simulink model "RA5_student"  (R2015b)
settings: Solver=ode1  StartTime=0.0  StopTime=1000  FixedStep=1/(1024*4)  RelTol=1e-3
settings Model: SimulationMode=external  Creator=root  LastModifiedBy=root
settings DataIOCC: LimitDataPoints=off  SaveFormat=Array  SignalLoggingSaveFormat=ModelDataLogs
settings OptimizationCC: ExpressionDepthLimit=2147483647  InitFltsAndDblsToZero=on
settings DebuggingCC: UnderspecifiedInitializationDetection=Classic  MergeDetectMultiDrivingBlocksExec=none  FcnCallInpInsideContextMsg=UseLocalSettings  UnconnectedInputMsg=none  UnconnectedOutputMsg=none  UnconnectedLineMsg=none  StateNameClashWarn=warning
settings HardwareCC: ProdBitPerPointer=32  ProdLargestAtomicFloat=None  ProdIntDivRoundTo=Undefined  ProdEndianess=Unspecified  ProdWordSize=32  ProdHWDeviceType=32-bit Generic
settings RTWCC: SystemTargetFile=ectarget.tlc  MakeCommand="make_rtw OPTS=\"-DNETIF_ID=2\""  TemplateMakefile=ec_unix.tmf  Description=EtherCAT Real-Time Target for SOEM  RTWVerbose=off  CustomInclude=/home/ebox/MATLAB/R2015b/toolbox/shapeit/
settings RTWCC: CustomSource=|
  | /home/ebox/MATLAB/R2015b/toolbox/shapeit/dleadlag.c
  | /home/ebox/MATLAB/R2015b/toolbox/shapeit/dlowpass2.c
  | /home/ebox/MATLAB/R2015b/toolbox/shapeit/dnotch.c
  | /home/ebox/MATLAB/R2015b/toolbox/shapeit/dpd.c
  | /home/ebox/MATLAB/R2015b/toolbox/shapeit/dweakint.c
settings GRTTargetCC: GeneratePreprocessorConditionals=Disable all  CombineOutputUpdateFcns=off  GRTInterface=on  UseToolchainInfoCompliant=off  ExtMode=on
settings ConfigComp: CovModelRefEnable=Off

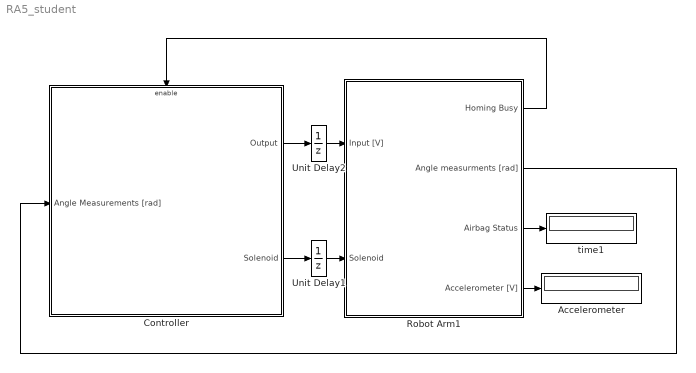
== system RA5_student ==
  Accelerometer : Display
      settings: Decimation=50
  Controller : Subsystem
  Robot Arm1 : Subsystem
      mask help: Simulink:masks:GenSFuncDesc_MD
      mask Help: eval('feval(''rtwprivate'',''rtwhelpview'',''rtw_sfcn_block'')');
      mask Display:
      | image(imread('RobotArm.png'))
      | color('red');port_label('output', 1, 'Homing Busy')
      | port_label('output', 2, 'Angle Measurements')
      | port_label('output', 3, 'Airbag Status')
      | port_label('output', 4, 'Accelerometer [V]')
      | port_label('input', 1, 'Input [V]')
      | port_label('input', 2, 'Solenoid')
  Unit Delay1 : UnitDelay  SampleTime=-1
  Unit Delay2 : UnitDelay  SampleTime=-1
  time1 : Display
      settings: Decimation=50
  wires:
  Controller/1(Output) -> Unit Delay2/1
  Robot Arm1/1(Homing Busy) -> Controller/Enable
  Robot Arm1/2(Angle measurments [rad]) -> Controller/1(Angle Measurements [rad])
  Robot Arm1/3(Airbag Status) -> time1/1
  Controller/2(Solenoid) -> Unit Delay1/1
  Robot Arm1/4(Accelerometer [V]) -> Accelerometer/1
  Unit Delay2/1 -> Robot Arm1/1(Input [V])
  Unit Delay1/1 -> Robot Arm1/2(Solenoid)

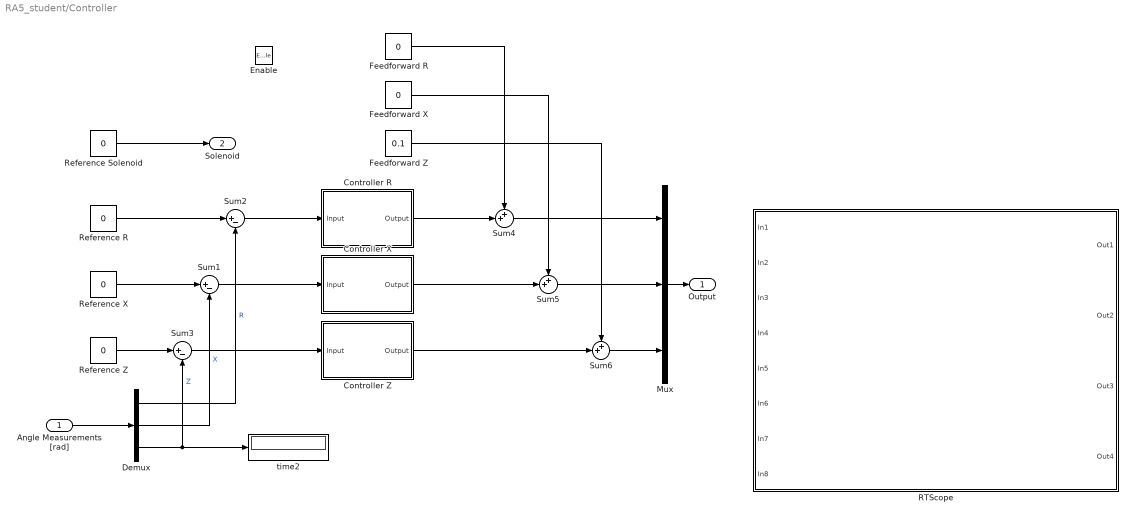
== system RA5_student/Controller ==
  Angle Measurements [rad] : Inport
  Enable : EnablePort
  Controller R : Subsystem
  Controller X : Subsystem
  Controller Z : Subsystem
  Demux : Demux  Outputs=3
  Feedforward R : Constant  Value=0
  Feedforward X : Constant  Value=0
  Feedforward Z : Constant  Value=0.1
  Mux : Mux  Inputs=3
  RTScope : Subsystem  mask(RTScope){}
      settings: OpenFcn=rtscope
      mask Display: image(imread('rtscope2.jpg'))
  Reference R : Constant  Value=0
  Reference Solenoid : Constant  Value=0
  Reference X : Constant  Value=0
  Reference Z : Constant  Value=0
  Sum1 : Sum  Inputs=|+-
  Sum2 : Sum  Inputs=|+-
  Sum3 : Sum  Inputs=|+-
  Sum4 : Sum  Inputs=++|  SaturateOnIntegerOverflow=on  InputSameDT=on  OutDataTypeStr=Inherit: Same as first input
  Sum5 : Sum  Inputs=++|  SaturateOnIntegerOverflow=on  InputSameDT=on  OutDataTypeStr=Inherit: Same as first input
  Sum6 : Sum  Inputs=++|  SaturateOnIntegerOverflow=on  InputSameDT=on  OutDataTypeStr=Inherit: Same as first input
  time2 : Display
      settings: Decimation=50
  Output : Outport
  Solenoid : Outport  Port=2  InitialOutput=0
  wires:
  Mux/1 -> Output/1
  Angle Measurements [rad]/1 -> Demux/1
  Sum2/1 -> Controller R/1(Input)
  Sum3/1 -> Controller Z/1(Input)
  Sum1/1 -> Controller X/1(Input)
  Demux/1 -> Sum2/2  "R"
  Demux/2 -> Sum1/2  "X"
  Demux/3 -> Sum3/2, time2/1  "Z"
  Feedforward R/1 -> Sum4/1
  Controller R/1(Output) -> Sum4/2
  Sum4/1 -> Mux/1
  Feedforward X/1 -> Sum5/1
  Controller X/1(Output) -> Sum5/2
  Sum5/1 -> Mux/2
  Controller Z/1(Output) -> Sum6/2
  Sum6/1 -> Mux/3
  Feedforward Z/1 -> Sum6/1
  Reference R/1 -> Sum2/1
  Reference X/1 -> Sum1/1
  Reference Z/1 -> Sum3/1
  Reference Solenoid/1 -> Solenoid/1

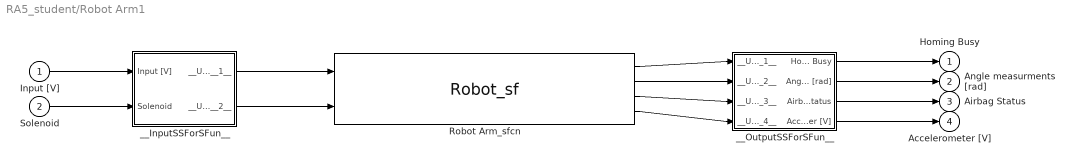
== system RA5_student/Robot Arm1 ==
  Input [V] : Inport
  Solenoid : Inport  Port=2
  Robot Arm_sfcn : S-Function  FunctionName=Robot_sf  SFunctionModules=dlowpass2 dnotch dpd dweakint ec_Ebox ec_EboxResetEnc  SFunctionDeploymentMode=off  EnableBusSupport=off  mask{rtw_sf_name=Robot_sf, showVar=off}
      mask prompts: rtw_sf_name "Simulink:masks:GenSFuncName_MP"; showVar "Simulink:masks:GenSFuncShowModuleList_MP"
      mask help: Simulink:masks:GenSFuncDesc_MD
      mask init:
      | displist = '';
      | if ~strcmp(get_param(gcb, 'FunctionName'), rtw_sf_name);
      |   set_param(gcb, 'FunctionName', rtw_sf_name);
      | end
      | % Check if we are generating code
      | rtw_mode = false;
      | if strcmpi(get_param(bdroot(gcb),'SimulationStatus'),'Initializing')
      | 	rtw_mode = strcmpi(get_param(bdroot(gcb),'BuildingRTWCode'),'on') && ...
      | 		~strcmpi(get_param(bdroot(gcb),'TargetStyle'),'SimulationTarget');
      | end
      | if showVar || rtw_mode
      | 	if exist('rtwsfunc') == 2 | exist('rtwsfunc') == 6
      | 		tmplist = rtwsfunc(rtw_sf_name,gcb);
      | 		tmplist = DAStudio.message('Simulink:masks:GenSFuncListOfModules_IC', tmplist);
      | 	elseif showVar
      | 		tmplist1 = DAStudio.message('Simulink:masks:GenSFuncListOfModules_IC', '');
      |         tmplist2 = DAStudio.message('Simulink:masks:GenSFuncNotLicensed_IC');
      |         tmplist = [tmplist1 tmplist2];
      |  	end
      | end
      | if showVar
      |   displist = tmplist;
      | end
      settings: CopyFcn=|
      | if ~strcmp(get_param(gcb,'Linkstatus'),'none') && ...
      | ~strcmp(get_param(gcb,'Linkstatus'),'implicit')
      |   set_param(gcb,'LinkStatus','none');
      | end
      mask Help: eval('feval(''rtwprivate'',''rtwhelpview'',''rtw_sfcn_block'')');
      mask Display:
      | port_label('input',1,'Input [V]');
      | port_label('input',2,'Solenoid');
      | port_label('output',1,'Homing Busy');
      | port_label('output',2,'Angle measurments [rad]');
      | port_label('output',3,'Airbag Status');
      | port_label('output',4,'Accelerometer [V]');
  __InputSSForSFun__ : Subsystem
  __OutputSSForSFun__ : Subsystem
  Homing Busy : Outport
  Angle measurments [rad] : Outport  Port=2
  Airbag Status : Outport  Port=3
  Accelerometer [V] : Outport  Port=4
  wires:
  __OutputSSForSFun__/4(Accelerometer [V]) -> Accelerometer [V]/1
  __OutputSSForSFun__/3(Airbag Status) -> Airbag Status/1
  __OutputSSForSFun__/2(Angle measurments [rad]) -> Angle measurments [rad]/1
  __OutputSSForSFun__/1(Homing Busy) -> Homing Busy/1
  Robot Arm_sfcn/4 -> __OutputSSForSFun__/4(__UniqueInportName__4__)
  Robot Arm_sfcn/3 -> __OutputSSForSFun__/3(__UniqueInportName__3__)
  Robot Arm_sfcn/2 -> __OutputSSForSFun__/2(__UniqueInportName__2__)
  Robot Arm_sfcn/1 -> __OutputSSForSFun__/1(__UniqueInportName__1__)
  __InputSSForSFun__/2(__UniqueOutportName__2__) -> Robot Arm_sfcn/2
  __InputSSForSFun__/1(__UniqueOutportName__1__) -> Robot Arm_sfcn/1
  Solenoid/1 -> __InputSSForSFun__/2(Solenoid)
  Input [V]/1 -> __InputSSForSFun__/1(Input [V])

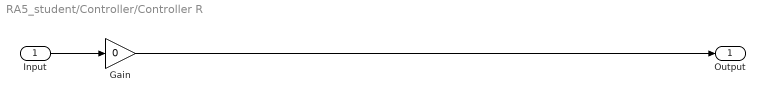
== system RA5_student/Controller/Controller R ==
  Input : Inport
  Gain : Gain  Gain=0
  Output : Outport
  wires:
  Input/1 -> Gain/1
  Gain/1 -> Output/1

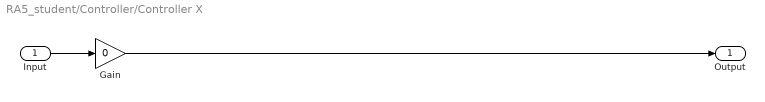
== system RA5_student/Controller/Controller X ==
  Input : Inport
  Gain : Gain  Gain=0
  Output : Outport
  wires:
  Gain/1 -> Output/1
  Input/1 -> Gain/1

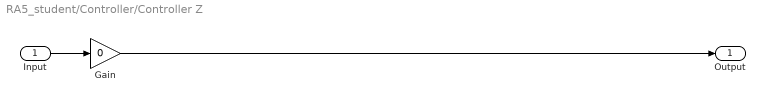
== system RA5_student/Controller/Controller Z ==
  Input : Inport
  Gain : Gain  Gain=0
  Output : Outport
  wires:
  Input/1 -> Gain/1
  Gain/1 -> Output/1

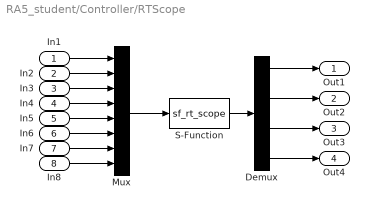
== system RA5_student/Controller/RTScope ==
  In1 : Inport
  In2 : Inport  Port=2
  In3 : Inport  Port=3
  In4 : Inport  Port=4
  In5 : Inport  Port=5
  In6 : Inport  Port=6
  In7 : Inport  Port=7
  In8 : Inport  Port=8
  Demux : Demux
  Mux : Mux  Inputs=8
  S-Function : S-Function  FunctionName=sf_rt_scope  Parameters=4096  SFunctionDeploymentMode=off  EnableBusSupport=off
  Out1 : Outport
  Out2 : Outport  Port=2
  Out3 : Outport  Port=3
  Out4 : Outport  Port=4
  wires:
  In8/1 -> Mux/8
  In7/1 -> Mux/7
  In6/1 -> Mux/6
  In5/1 -> Mux/5
  In4/1 -> Mux/4
  In3/1 -> Mux/3
  In2/1 -> Mux/2
  In1/1 -> Mux/1
  Demux/4 -> Out4/1
  Demux/3 -> Out3/1
  Demux/2 -> Out2/1
  Demux/1 -> Out1/1
  S-Function/1 -> Demux/1
  Mux/1 -> S-Function/1

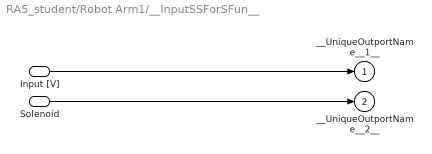
== system RA5_student/Robot Arm1/__InputSSForSFun__ ==
  Input [V] : Inport
  Solenoid : Inport  Port=2
  __UniqueOutportName__1__ : Outport
  __UniqueOutportName__2__ : Outport  Port=2
  wires:
  Solenoid/1 -> __UniqueOutportName__2__/1
  Input [V]/1 -> __UniqueOutportName__1__/1

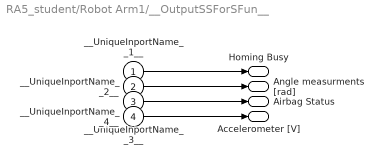
== system RA5_student/Robot Arm1/__OutputSSForSFun__ ==
  __UniqueInportName__1__ : Inport
  __UniqueInportName__2__ : Inport  Port=2
  __UniqueInportName__3__ : Inport  Port=3
  __UniqueInportName__4__ : Inport  Port=4
  Homing Busy : Outport
  Angle measurments [rad] : Outport  Port=2
  Airbag Status : Outport  Port=3
  Accelerometer [V] : Outport  Port=4
  wires:
  __UniqueInportName__4__/1 -> Accelerometer [V]/1
  __UniqueInportName__3__/1 -> Airbag Status/1
  __UniqueInportName__2__/1 -> Angle measurments [rad]/1
  __UniqueInportName__1__/1 -> Homing Busy/1
